simulink model "Pb_2"  (R2020b)
settings: Solver=VariableStepAuto  StartTime=0.0  StopTime=100  RelTol=1e-3
values from neighbouring files (symbols this model uses):
  b1 = 350    [Problem_2.m]
  k1 = 50000    [Problem_2.m]
  k2 = 50000    [Problem_2.m]
  m1 = 2500    [Problem_2.m]
  m2 = 320    [Problem_2.m]
settings Model: Creator=Ganesh  LastModifiedBy=Hinal
settings DataIOCC: ExternalInput=[t, stin]  LoadExternalInput=on  SaveFormat=Structure

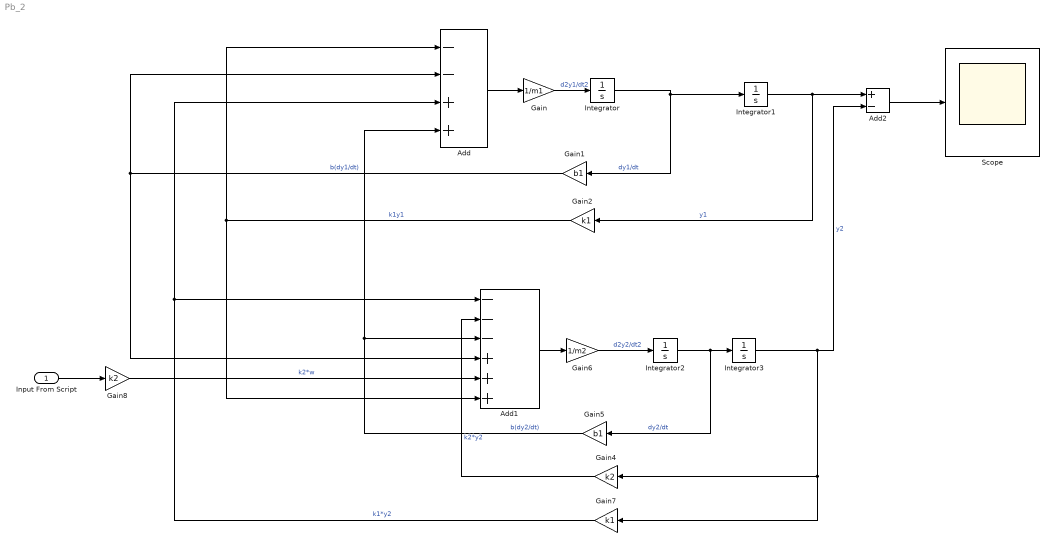
== system Pb_2 ==
  Input From Script : Inport
  Add : Sum  Inputs=--++
  Add1 : Sum  Inputs=---+++
  Add2 : Sum  Inputs=+-
  Gain : Gain  Gain=1/m1
  Gain1 : Gain  Gain=b1
  Gain2 : Gain  Gain=k1
  Gain4 : Gain  Gain=k2
  Gain5 : Gain  Gain=b1
  Gain6 : Gain  Gain=1/m2
  Gain7 : Gain  Gain=k1
  Gain8 : Gain  Gain=k2
  Integrator{,1..3} (4 alike) : Integrator
  Scope : Scope
  wires:
  Add/1 -> Gain/1
  Gain/1 -> Integrator/1  "d2y1/dt2"
  Integrator/1 -> Integrator1/1, Gain1/1  "dy1/dt"
  Integrator1/1 -> Add2/1, Gain2/1  "y1"
  Gain1/1 -> Add/2, Add1/4  "b(dy1/dt)"
  Add1/1 -> Gain6/1
  Gain6/1 -> Integrator2/1  "d2y2/dt2"
  Integrator2/1 -> Gain5/1, Integrator3/1  "dy2/dt"
  Integrator3/1 -> Gain7/1, Gain4/1, Add2/2  "y2"
  Gain4/1 -> Add1/2  "k2*y2"
  Gain5/1 -> Add/4, Add1/3  "b(dy2/dt)"
  Gain7/1 -> Add/3, Add1/1  "k1*y2"
  Input From Script/1 -> Gain8/1
  Gain2/1 -> Add/1, Add1/6  "k1y1"
  Gain8/1 -> Add1/5  "k2*w"
  Add2/1 -> Scope/1
